simulink library "BumplessPID_Lib"  (R2020a)
settings: Solver=VariableStepAuto  StartTime=0.0  StopTime=10.0  RelTol=1e-3
libraries: simulink x1
settings Model: Creator=Christian  LastModifiedBy=Christian

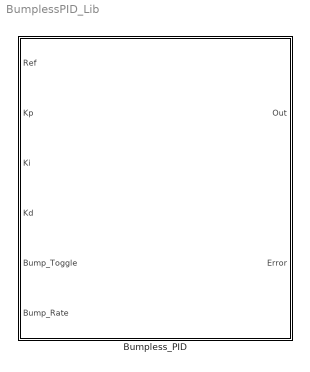
== system BumplessPID_Lib ==
  Bumpless_PID : Subsystem

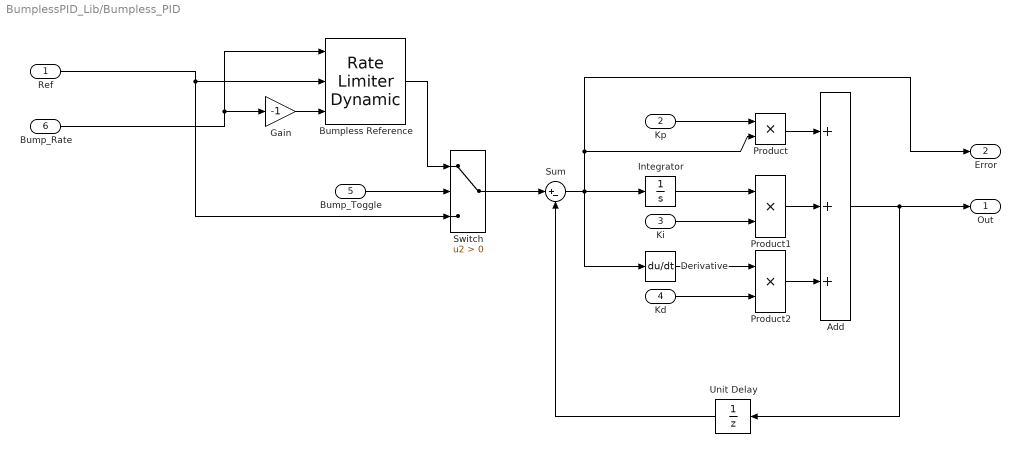
== system BumplessPID_Lib/Bumpless_PID ==
  Ref : Inport
  Kp : Inport  Port=2
  Ki : Inport  Port=3
  Kd : Inport  Port=4
  Bump_Toggle : Inport  Port=5
  Bump_Rate : Inport  Port=6
  Add : Sum  Inputs=+++
  Bumpless Reference : simulink/Discontinuities/Rate Limiter Dynamic
  Derivative : Derivative
  Gain : Gain  Gain=-1
  Integrator : Integrator
  Product : Product
  Product1 : Product
  Product2 : Product
  Sum : Sum  Inputs=|+-
  Switch : Switch  Criteria=u2 > Threshold
  Unit Delay : UnitDelay  SampleTime=-1  HasFrameUpgradeWarning=on
  Out : Outport
  Error : Outport  Port=2
  wires:
  Bump_Toggle/1 -> Switch/2
  Ref/1 -> Switch/3, Bumpless Reference/2
  Bumpless Reference/1 -> Switch/1
  Bump_Rate/1 -> Gain/1, Bumpless Reference/1
  Gain/1 -> Bumpless Reference/3
  Switch/1 -> Sum/1
  Kp/1 -> Product/1
  Product/1 -> Add/1
  Ki/1 -> Product1/2
  Product1/1 -> Add/2
  Kd/1 -> Product2/2
  Sum/1 -> Error/1, Product/2, Integrator/1, Derivative/1
  Product2/1 -> Add/3
  Add/1 -> Unit Delay/1, Out/1
  Unit Delay/1 -> Sum/2
  Derivative/1 -> Product2/1
  Integrator/1 -> Product1/1
